simulink library "CHU_FSAE_BMS_Lib"  (R2025b)
settings: Solver=VariableStepAuto  StartTime=0.0  StopTime=10.0  RelTol=1e-3
settings Model: Creator=Admin1  LastModifiedBy=Admin1

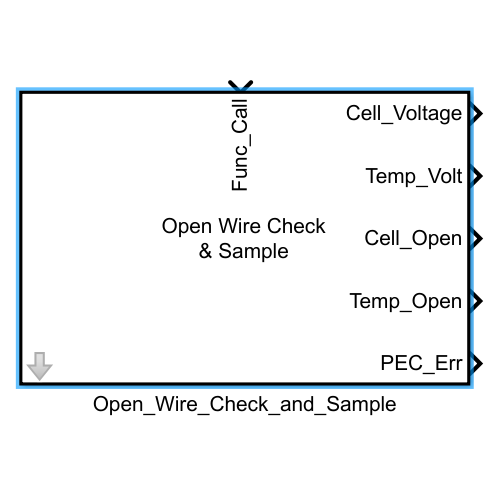
[thumbnail: Simulink's stored preview of the top-level diagram]
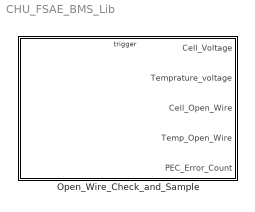
== system CHU_FSAE_BMS_Lib ==
  Open_Wire_Check_and_Sample : Subsystem  TreatAsAtomicUnit=on
      mask DialogControl ParameterGroupVar Prompt: 参数
      mask Display:
      | disp('Open Wire Check\n& Sample');
      | port_label('input',1,'Func_Call');
      | port_label('output',1,'Cell_Voltage');
      | port_label('output',2,'Temp_Volt');
      | port_label('output',3,'Cell_Open');
      | port_label('output',4,'Temp_Open');
      | port_label('output',5,'PEC_Err');

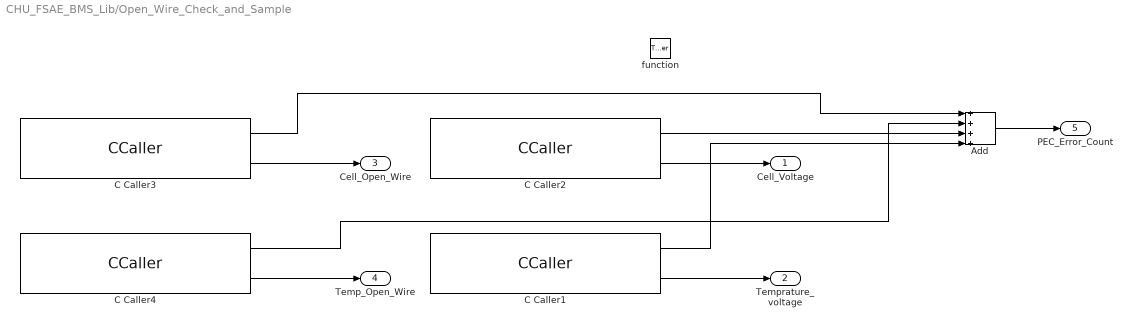
== system CHU_FSAE_BMS_Lib/Open_Wire_Check_and_Sample ==
  function : TriggerPort  TriggerType=function-call  VariantControl=(inherit)  SampleTimeType=periodic  SampleTime=0.01
  Add : Sum  Inputs=++++
  C Caller1 : CCaller  Priority=3  FunctionName=Bms_SampleTemperature  PortSpecificationStruct="%)30     .    R ,   8    (     @         %    \"     (    !     0         %  0 \"0    $    _    07)G3F%M90  4&]R=$YA;64 4V-O<&4     26YD97@     5'EP90      4VEZ90      27-';&]B86P   X    P    !@    @    $          4    (     0    ,    !         !   P!O=70 #@   #     &    \"     0         !0    @    !     P    $         $  # &]U=  .    .     8    (    !          %    \"     $    &     0         0    !@   $]U='!U=   #@   #@    &    \"     8         !0    @    !     0    $         \"0    @               X    X    !@    @    $          4    (     0    4    !         !     %    =6EN=#@    .    ,     8    (    !          %    \"     $    !     0         0  $ ,0    X    P    !@    @    ) @        4    (     0    $    !          (  0      #@   #@    &    \"     0         !0    @    !    !0    $         $     4   !C;V1E<P    X    X    !@    @    $          4    (     0    4    !         !     %    8V]D97,    .    .     8    (    !          %    \"     $    &     0         0    !@   $]U='!U=   #@   #@    &    \"     8         !0    @    !     0    $         \"0    @           #P/PX    X    !@    @    $          4    (     0    8    !         !     &    =6EN=#$V   .    ,     8    (    !          %    \"     $    \"     0         0  ( -30   X    P    !@    @    ) @        4    (     0    $    !          (  0"
  C Caller2 : CCaller  Priority=2  FunctionName=Bms_SampleCellVoltage  PortSpecificationStruct="%)30     .    R ,   8    (     @         %    \"     (    !     0         %  0 \"0    $    _    07)G3F%M90  4&]R=$YA;64 4V-O<&4     26YD97@     5'EP90      4VEZ90      27-';&]B86P   X    P    !@    @    $          4    (     0    ,    !         !   P!O=70 #@   #     &    \"     0         !0    @    !     P    $         $  # &]U=  .    .     8    (    !          %    \"     $    &     0         0    !@   $]U='!U=   #@   #@    &    \"     8         !0    @    !     0    $         \"0    @               X    X    !@    @    $          4    (     0    4    !         !     %    =6EN=#@    .    ,     8    (    !          %    \"     $    !     0         0  $ ,0    X    P    !@    @    ) @        4    (     0    $    !          (  0      #@   #@    &    \"     0         !0    @    !    !0    $         $     4   !C;V1E<P    X    X    !@    @    $          4    (     0    4    !         !     %    8V]D97,    .    .     8    (    !          %    \"     $    &     0         0    !@   $]U='!U=   #@   #@    &    \"     8         !0    @    !     0    $         \"0    @           #P/PX    X    !@    @    $          4    (     0    8    !         !     &    =6EN=#$V   .    ,     8    (    !          %    \"     $    #     0         0  , ,3 X  X    P    !@    @    ) @        4    (     0    $    !          (  0"
  C Caller3 : CCaller  Priority=0  FunctionName=Bms_DetectCellOpenWire  PortSpecificationStruct="%)30     .    R ,   8    (     @         %    \"     (    !     0         %  0 \"0    $    _    07)G3F%M90  4&]R=$YA;64 4V-O<&4     26YD97@     5'EP90      4VEZ90      27-';&]B86P   X    P    !@    @    $          4    (     0    ,    !         !   P!O=70 #@   #     &    \"     0         !0    @    !     P    $         $  # &]U=  .    .     8    (    !          %    \"     $    &     0         0    !@   $]U='!U=   #@   #@    &    \"     8         !0    @    !     0    $         \"0    @               X    X    !@    @    $          4    (     0    4    !         !     %    =6EN=#@    .    ,     8    (    !          %    \"     $    !     0         0  $ ,0    X    P    !@    @    ) @        4    (     0    $    !          (  0      #@   #@    &    \"     0         !0    @    !    !0    $         $     4   !F;&%G<P    X    X    !@    @    $          4    (     0    4    !         !     %    9FQA9W,    .    .     8    (    !          %    \"     $    &     0         0    !@   $]U='!U=   #@   #@    &    \"     8         !0    @    !     0    $         \"0    @           #P/PX    X    !@    @    $          4    (     0    4    !         !     %    =6EN=#@    .    ,     8    (    !          %    \"     $    #     0         0  , ,3$T  X    P    !@    @    ) @        4    (     0    $    !          (  0"
  C Caller4 : CCaller  Priority=1  FunctionName=Bms_DetectTempOpenWire  PortSpecificationStruct="%)30     .    R ,   8    (     @         %    \"     (    !     0         %  0 \"0    $    _    07)G3F%M90  4&]R=$YA;64 4V-O<&4     26YD97@     5'EP90      4VEZ90      27-';&]B86P   X    P    !@    @    $          4    (     0    ,    !         !   P!O=70 #@   #     &    \"     0         !0    @    !     P    $         $  # &]U=  .    .     8    (    !          %    \"     $    &     0         0    !@   $]U='!U=   #@   #@    &    \"     8         !0    @    !     0    $         \"0    @               X    X    !@    @    $          4    (     0    4    !         !     %    =6EN=#@    .    ,     8    (    !          %    \"     $    !     0         0  $ ,0    X    P    !@    @    ) @        4    (     0    $    !          (  0      #@   #@    &    \"     0         !0    @    !    !0    $         $     4   !F;&%G<P    X    X    !@    @    $          4    (     0    4    !         !     %    9FQA9W,    .    .     8    (    !          %    \"     $    &     0         0    !@   $]U='!U=   #@   #@    &    \"     8         !0    @    !     0    $         \"0    @           #P/PX    X    !@    @    $          4    (     0    4    !         !     %    =6EN=#@    .    ,     8    (    !          %    \"     $    \"     0         0  ( -30   X    P    !@    @    ) @        4    (     0    $    !          (  0"
  Cell_Voltage : Outport
  Temprature_voltage : Outport  Port=2
  Cell_Open_Wire : Outport  Port=3
  Temp_Open_Wire : Outport  Port=4
  PEC_Error_Count : Outport  Port=5
  wires:
  C Caller2/2 -> Cell_Voltage/1
  C Caller1/2 -> Temprature_voltage/1
  C Caller3/2 -> Cell_Open_Wire/1
  C Caller4/2 -> Temp_Open_Wire/1
  C Caller3/1 -> Add/1
  C Caller4/1 -> Add/2
  C Caller2/1 -> Add/3
  C Caller1/1 -> Add/4
  Add/1 -> PEC_Error_Count/1
